simulink model "souk_single_pipeline_4x2"  (R2021a)
settings: Solver=VariableStepAuto  StartTime=0.0  StopTime=10.0  RelTol=1e-3
undefined symbols (not defined in the file): datetime, posixtime
libraries: xbsIndex_r4 x9016, casper_library_misc x75, casper_library_delays x33, casper_library_reorder x22, xps_library x10
(part 73 of 104)

== system souk_single_pipeline_4x2/p0/synth_input_reorder1/map0/map1 ==
  addr : Inport
  data_in : Inport  Port=2
  we : Inport  Port=3
  Terminator : Terminator
  Terminator1 : Terminator
  Terminator2 : Terminator
  calc_add : Subsystem  mask{data_width=32, addr_width=12, sample_rate=sample_rate}
      mask prompts: data_width "data width"; addr_width "address width"; sample_rate "sample rate"
  convert_addr : xbsIndex_r4/Convert  gui_display_data_type=Fixed-point  arith_type=Unsigned  n_bits=addr_width  bin_pt=0  float_type=Single  exp_bits=8  fraction_bits=24  quantization=Truncate  overflow=Wrap  en=off  latency=0  pipeline=off  dbl_ovrd=off  block_type=convert
      settings: xl_area=[0, 0, 0, 0, 0, 0, 0]
  convert_din1 : xbsIndex_r4/Convert  gui_display_data_type=Fixed-point  arith_type=Unsigned  n_bits=32  bin_pt=0  float_type=Single  exp_bits=8  fraction_bits=24  quantization=Truncate  overflow=Wrap  en=off  latency=0  pipeline=off  dbl_ovrd=off  block_type=convert
      settings: xl_area=[0, 0, 0, 0, 0, 0, 0]
  convert_we : xbsIndex_r4/Convert  gui_display_data_type=Fixed-point  arith_type=Unsigned  n_bits=1  bin_pt=0  float_type=Single  exp_bits=8  fraction_bits=24  quantization=Truncate  overflow=Wrap  en=off  latency=0  pipeline=off  dbl_ovrd=off  block_type=convert
      settings: xl_area=[0, 0, 0, 0, 0, 0, 0]
  munge_in : Subsystem  AncestorBlock=casper_library_flow_control/munge  mask(munge){divisions=1, div_size=32, order=[0], arith_type_out=Unsigned, bin_pt_out=0}
      mask prompts: divisions "Number of divisions"; div_size "Division size (bits)"; order "Division packing order"; arith_type_out "Output arithmetic type"; bin_pt_out "Output binary point"
      mask help: Splits an input bus into the specified number of divisions and then recombines them in the order specified (most significant division = 0,least = number divisions-1)
      mask init:
      | munge_init(gcb, ...
      |     'divisions', divisions, ...
      |     'div_size', div_size, ...
      |     'order', order, ...
      |     'arith_type_out', arith_type_out, ...
      |     'bin_pt_out', bin_pt_out);
      settings: AttributesFormatString=|
      | split:32
      | join:0
      | Unsigned [32,0]
      mask TypeOptions arith_type_out: Unsigned | Signed  (2's comp) | Floating-point
  munge_out : Subsystem  AncestorBlock=casper_library_flow_control/munge  mask(munge){divisions=1, div_size=32, order=[0], arith_type_out=Unsigned, bin_pt_out=0}
      mask prompts: divisions "Number of divisions"; div_size "Division size (bits)"; order "Division packing order"; arith_type_out "Output arithmetic type"; bin_pt_out "Output binary point"
      mask help: Splits an input bus into the specified number of divisions and then recombines them in the order specified (most significant division = 0,least = number divisions-1)
      mask init:
      | munge_init(gcb, ...
      |     'divisions', divisions, ...
      |     'div_size', div_size, ...
      |     'order', order, ...
      |     'arith_type_out', arith_type_out, ...
      |     'bin_pt_out', bin_pt_out);
      settings: AttributesFormatString=|
      | split:32
      | join:0
      | Unsigned [32,0]
      mask TypeOptions arith_type_out: Unsigned | Signed  (2's comp) | Floating-point
  sim_mem : Subsystem  mask{arith_type=Unsigned, addr_width=12, data_width=32, data_bin_pt=0, init_vals=[4095  4094  4093  4092  4091  4090  4089  4088  4087  4086  4085  4084  4083  4082  4081  4080  4079  4078  4077  4076  4075  4074  4073  4072  4071  4070  4069  4068  4067  4066  4065  4064  4063  4062  4061  4060  4059  4058  4057  4056  4055  4054  4053  4052  4051  4050  4049  4048  4047  4046  4045  4044  4043  4042  4041  4040  4039  4038  4037  4036  4035  4034  4033  4032  4031  4030  4029  4028  4027  4026  4025  4024  4023  4022  4021  4020  4019  4018  4017  4016  4015  4014  4013  4012  4011  4010  4009  4008  4007  4006  4005  4004  4003  4002  4001  4000  3999  3998  3997  3996  3995  3994  3993  3992  3991  3990  3989  3988  3987  3986  3985  3984  3983  3982  3981  3980  3979  3978  3977  3976  3975  3974  3973  3972  3971  3970  3969  3968  3967  3966  3965  3964  3963  3962  3961  3960  3959  3958  3957  3956  3955  3954  3953  3952  3951  3950  3949  3948  3947  3946  3945  3944  3943  3942  3941  3940  3939  3938  3937  3936  3935  3934  3933  3932  3931  3930  3929  3928  3927  3926  3925  3924  3923  3922  3921  3920  3919  3918  3917  3916  3915  3914  3913  3912  3911  3910  3909  3908  3907  3906  3905  3904  3903  3902  3901  3900  3899  3898  3897  3896  3895  3894  3893  3892  3891  3890  3889  3888  3887  3886  3885  3884  3883  3882  3881  3880  3879  3878  3877  3876  3875  3874  3873  3872  3871  3870  3869  3868  3867  3866  3865  3864  3863  3862  3861  3860  3859  3858  3857  3856  3855  3854  3853  3852  3851  3850  3849  3848  3847  3846  3845  3844  3843  3842  3841  3840  3839  3838  3837  3836  3835  3834  3833  3832  3831  3830  3829  3828  3827  3826  3825  3824  3823  3822  3821  3820  3819  3818  3817  3816  3815  3814  3813  3812  3811  3810  3809  3808  3807  3806  3805  3804  3803  3802  3801  3800  3799  3798  3797  3796  3795  3794  3793  3792  3791  3790  3789  3788  3787  3786  3785  3784  3783  3782  3781  3780  3779  3778  3777  3776  3775  3774  3773  3772  3771  3770  3769  3768  3767  3766  3765  3764  3763  3762  3761  3760  3759  3758  3757  3756  3755  3754  3753  3752  3751  3750  3749  3748  3747  3746  3745  3744  3743  3742  3741  3740  3739  3738  3737  3736  3735  3734  3733  3732  3731  3730  3729  3728  3727  3726  3725  3724  3723  3722  3721  3720  3719  3718  3717  3716  3715  3714  3713  3712  3711  3710  3709  3708  3707  3706  3705  3704  3703  3702  3701  3700  3699  3698  3697  3696  3695  3694  3693  3692  3691  3690  3689  3688  3687  3686  3685  3684  3683  3682  3681  3680  3679  3678  3677  3676  3675  3674  3673  3672  3671  3670  3669  3668  3667  3666  3665  3664  3663  3662  3661  3660  3659  3658  3657  3656  3655  3654  3653  3652  3651  3650  3649  3648  3647  3646  3645  3644  3643  3642  3641  3640  3639  3638  3637  3636  3635  3634  3633  3632  3631  3630  3629  3628  3627  3626  3625  3624  3623  3622  3621  3620  3619  3618  3617  3616  3615  3614  3613  3612  3611  3610  3609  3608  3607  3606  3605  3604  3603  3602  3601  3600  3599  3598  3597  3596  3595  3594  3593  3592  3591  3590  3589  3588  3587  3586  3585  3584  3583  3582  3581  3580  3579  3578  3577  3576  3575  3574  3573  3572  3571  3570  3569  3568  3567  3566  3565  3564  3563  3562  3561  3560  3559  3558  3557  3556  3555  3554  3553  3552  3551  3550  3549  3548  3547  3546  3545  3544  3543  3542  3541  3540  3539  3538  3537  3536  3535  3534  3533  3532  3531  3530  3529  3528  3527  3526  3525  3524  3523  3522  3521  3520  3519  3518  3517  3516  3515  3514  3513  3512  3511  3510  3509  3508  3507  3506  3505  3504  3503  3502  3501  3500  3499  3498  3497  3496  3495  3494  3493  3492  3491  3490  3489  3488  3487  3486  3485  3484  3483  3482  3481  3480  3479  3478  3477  3476  3475  3474  3473  3472  3471  3470  3469  3468  3467  3466  3465  3464  3463  3462  3461  3460  3459  3458  3457  3456  3455  3454  3453  3452  3451  3450  3449  3448  3447  3446  3445  3444  3443  3442  3441  3440  3439  3438  3437  3436  3435  3434  3433  3432  3431  3430 ...(+20579 chars)], sample_rate=1, csp_latency=1}
      mask prompts: arith_type "Output Data Type"; addr_width "Address width"; data_width "Data width"; data_bin_pt "Data Binary Point"; init_vals "Initial values"; sample_rate "Sample rate"; csp_latency "Latency"
      mask init:
      | % set_param([gcb, '/data_to_xilinx'], 'arith_type', arith_type)
      | % set_param([gcb, '/data_to_xilinx'], 'n_bits', get_param(gcb, 'data_width'))
      mask TypeOptions arith_type: Unsigned | Signed  (2's comp)
      mask TypeOptions data_width: 8 | 16 | 32 | 64 | 128 | 256 | 512 | 1024
  souk_single_pipeline_krm_p0_synth_input_reorder1_map0_map1_addr : xbsIndex_r4/Gateway Out  inherit_from_input=off  hdl_port=on  rows=1  columns=1  UseAsDAC=off  DACChannel='1'  interface=None  automatic_assignment=on  address_offset=hex2dec('00')  intf_name=''  intf_description=''  timing_constraint=None  locs_specified=off  LOCs={'A5','B9','A9','C1','A3','G6','E9','A6','A7','A8','B8','B1','B3','D9','B5','B4','B6','C2'}  io_standard={}  block_type=gatewayout
      settings: infoedit="Gateway out block.  Converts Xilinx fixed point inputs into ouputs of type Simulink integer, double, or fixed point.<P><P>Hardware notes:  In hardware these blocks become top level output ports or are discarded, depending on how they are configured."  sginterface={'Nallatech'=>{'xdspkit'=>{'non_memory_mapped_port'=>'uprev_Shared_BRAM_addr'}},'Xilinx'=>{'jtaghwcosim'=>{'non_memory_mapped_port'=>'uprev_Shared_BRAM_addr'},'xdspkit'=>{'non_memory_mapped_port'=>'uprev_Shared_BRAM_addr'}}}  xl_area=[0, 0, 0, 0, 0, 0, 0]
  souk_single_pipeline_krm_p0_synth_input_reorder1_map0_map1_data_in : xbsIndex_r4/Gateway Out  inherit_from_input=off  hdl_port=on  rows=1  columns=1  UseAsDAC=off  DACChannel='1'  interface=None  automatic_assignment=on  address_offset=hex2dec('00')  intf_name=''  intf_description=''  timing_constraint=None  locs_specified=off  LOCs={'B21','B22','A22','B23','B19','C19','A20','A21','A23','B24','A24','A25','E18','D18','C18','B18'}  io_standard={}  block_type=gatewayout
      settings: infoedit="Gateway out block.  Converts Xilinx fixed point inputs into ouputs of type Simulink integer, double, or fixed point.<P><P>Hardware notes:  In hardware these blocks become top level output ports or are discarded, depending on how they are configured."  sginterface={'Nallatech'=>{'xdspkit'=>{'non_memory_mapped_port'=>'uprev_Shared_BRAM_data_in'}},'Xilinx'=>{'jtaghwcosim'=>{'non_memory_mapped_port'=>'uprev_Shared_BRAM_data_in'},'xdspkit'=>{'non_memory_mapped_port'=>'uprev_Shared_BRAM_data_in'}}}  xl_area=[0, 0, 0, 0, 0, 0, 0]
  souk_single_pipeline_krm_p0_synth_input_reorder1_map0_map1_data_out : xbsIndex_r4/Gateway In  gui_display_data_type=Fixed-point  arith_type=Unsigned  n_bits=32  bin_pt=0  preci_type=Single  exp_width=8  frac_width=24  rows=1  columns=1  quantization=Truncate  overflow=Wrap  period=sample_rate  UseAsADC=off  ADCChannel='1'  interface=None  automatic_assignment=on  address_offset=hex2dec('00')  intf_name=''  intf_description=''  default_value=0  timing_constraint=None  locs_specified=off  LOCs={}  io_standard={}  inherit_from_input=off  hdl_port=on  dbl_ovrd=off  block_type=gatewayin
      settings: xl_area=[0, 0, 0, 0, 0, 0, 0]
  souk_single_pipeline_krm_p0_synth_input_reorder1_map0_map1_we : xbsIndex_r4/Gateway Out  inherit_from_input=off  hdl_port=on  rows=1  columns=1  UseAsDAC=off  DACChannel='1'  interface=None  automatic_assignment=on  address_offset=hex2dec('00')  intf_name=''  intf_description=''  timing_constraint=None  locs_specified=off  LOCs={'A14'}  io_standard={}  block_type=gatewayout
      settings: infoedit="Gateway out block.  Converts Xilinx fixed point inputs into ouputs of type Simulink integer, double, or fixed point.<P><P>Hardware notes:  In hardware these blocks become top level output ports or are discarded, depending on how they are configured."  xl_area=[0, 0, 0, 0, 0, 0, 0]
  data_out : Outport  VectorParamsAs1DForOutWhenUnconnected=off
  wires:
  munge_out/1(dout) -> data_out/1
  sim_mem/1(data_out) -> souk_single_pipeline_krm_p0_synth_input_reorder1_map0_map1_data_out/1
  souk_single_pipeline_krm_p0_synth_input_reorder1_map0_map1_data_out/1 -> munge_out/1(din)
  convert_addr/1 -> souk_single_pipeline_krm_p0_synth_input_reorder1_map0_map1_addr/1
  convert_din1/1 -> souk_single_pipeline_krm_p0_synth_input_reorder1_map0_map1_data_in/1
  data_in/1 -> munge_in/1(din)
  calc_add/1(out) -> convert_addr/1
  souk_single_pipeline_krm_p0_synth_input_reorder1_map0_map1_we/1 -> Terminator2/1
  souk_single_pipeline_krm_p0_synth_input_reorder1_map0_map1_data_in/1 -> Terminator1/1
  souk_single_pipeline_krm_p0_synth_input_reorder1_map0_map1_addr/1 -> Terminator/1
  convert_we/1 -> souk_single_pipeline_krm_p0_synth_input_reorder1_map0_map1_we/1
  addr/1 -> sim_mem/1(addr), calc_add/1(in)
  we/1 -> sim_mem/3(we), convert_we/1
  munge_in/1(dout) -> sim_mem/2(data), convert_din1/1

== system souk_single_pipeline_4x2/p0/synth_input_reorder1/map0/we_expand ==
  bus_in : Inport
  slice1 : xbsIndex_r4/Slice  nbits=1  boolean_output=on  mode=Upper Bit Location + Width  bit1=0  base1=MSB of Input  bit0=0  base0=LSB of Input  dbl_ovrd=off  block_type=slice
  msb_lsb_out1 : Outport
  wires:
  bus_in/1 -> slice1/1
  slice1/1 -> msb_lsb_out1/1

== system souk_single_pipeline_4x2/p0/synth_input_reorder1/map0/we_replicate ==
  in : Inport
  bussify : Subsystem  AncestorBlock=casper_library_flow_control/bus_create  mask(bus_create){inputNum=1}
      mask prompts: inputNum "Number of inputs:"
      mask init:
      | bus_create_init(gcb,...
      |     'inputNum', inputNum);
  out : Outport
  wires:
  in/1 -> bussify/1(in1)
  bussify/1(bus_out) -> out/1

== system souk_single_pipeline_4x2/p0/synth_input_reorder1/map1/addr_expand ==
  bus_in : Inport
  reinterpret1 : xbsIndex_r4/Reinterpret  force_arith_type=on  arith_type=Unsigned  force_bin_pt=on  bin_pt=0  block_type=reinterpret
  slice1 : xbsIndex_r4/Slice  nbits=12  boolean_output=off  mode=Upper Bit Location + Width  bit1=0  base1=MSB of Input  bit0=0  base0=LSB of Input  dbl_ovrd=off  block_type=slice
  msb_lsb_out1 : Outport
  wires:
  bus_in/1 -> slice1/1
  slice1/1 -> reinterpret1/1
  reinterpret1/1 -> msb_lsb_out1/1

== system souk_single_pipeline_4x2/p0/synth_input_reorder1/map1/addr_replicate ==
  in : Inport
  bussify : Subsystem  AncestorBlock=casper_library_flow_control/bus_create  mask(bus_create){inputNum=1}
      mask prompts: inputNum "Number of inputs:"
      mask init:
      | bus_create_init(gcb,...
      |     'inputNum', inputNum);
  out : Outport
  wires:
  bussify/1(bus_out) -> out/1
  in/1 -> bussify/1(in1)
